simulink model "Monza_simulacion"  (R2023b)
settings: Solver=VariableStepAuto  StartTime=0.0  StopTime=20  RelTol=1e-3
values from neighbouring files (symbols this model uses):
  Ts = 0.005    [simulacion_monza_tfm.m]
libraries: slpidlib x2
settings Model: PauseTimes=20  Creator=christian  LastModifiedBy=Usuario
settings SolverCC: ZeroCrossAlgorithm=Adaptive  AlgebraicLoopSolver=TrustRegion
settings DataIOCC: ReturnWorkspaceOutputs=off
settings DebuggingCC: UnconnectedInputMsg=warning  UnconnectedOutputMsg=warning  UnconnectedLineMsg=warning  ArithmeticOperatorsInVariantConditions=warning
settings ModelReferenceCC: EnableRefExpFcnMdlSchedulingChecks=on
settings SFSimCC: SimUseLocalCustomCode=off  CustomCodeUndefinedFunction=UseInterfaceOnly
settings RTWCC: RTWUseLocalCustomCode=off

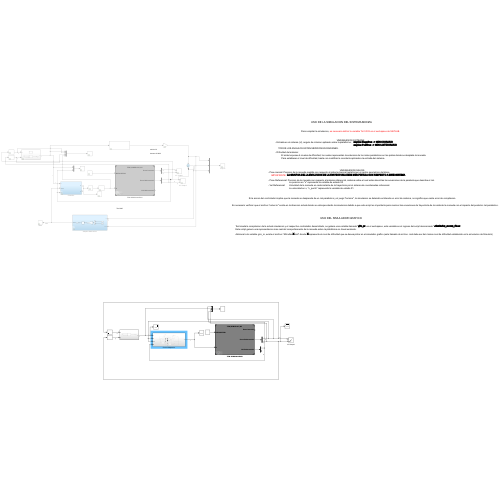
[thumbnail: Simulink's stored preview of the top-level diagram]
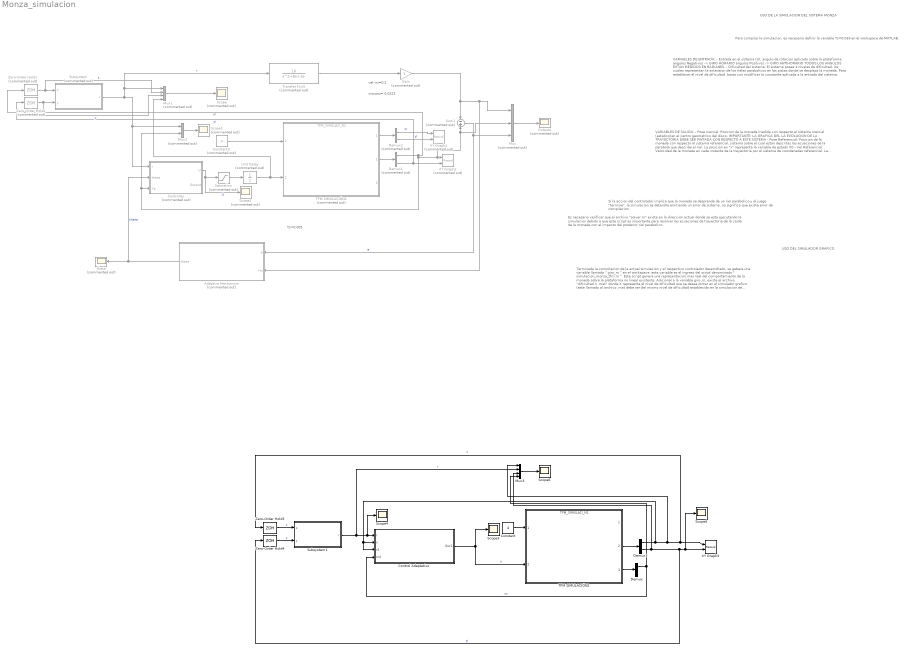
== system Monza_simulacion ==
  note: viscoso= 0.0223
  note: vel-ini=0.2
  note: Ts=0.005
  note: Es necesario verificar que el archivo "solver.m" exista en la direccion actual donde se esta ejecutando la simulacion debido a que este script es importante para resolver las ecuaciones de trayectoria de la caida de la moneda con el impacto del posterior riel parabolico.
  note: Si la accion del controlador implica que la moneda se desprenda de un riel parabolico y el juego "termine", la simulacion se detendra emitiendo un error de sistema, no significa que existe error de compilacion.
  note: Para compilar la simulacion, es necesario definir la variable Ts=0.033 en el workspace de MATLAB.
  note: VARIABLES DE ENTRADA:
      | - Entrada en el sistema (U), angulo de rotacion aplicado sobre la plataforma; angulos Negativos -> GIRO HORARIO
      | angulos Positivos -> GIRO ANTIHORARIO
      | TODOS LOS ANGULOS ESTAN MEDIDOS EN RADIANES.
      |
      | - Dificultad del sistema:
      | El sistema posee 4 niveles de dificultad, los cuales representan la extension de los rieles parabolicos en las pistas donde se desplaza la moneda.
      | Para establecer el nivel de dificultad, basta con modificar la constante aplicada a la entrada del sistema.
  note: USO DE LA SIMULACION DEL SISTEMA MONZA
  note: VARIABLES DE SALIDA:
      | - Pose inercial: Posicion de la moneda medida con respecto al sistema Inercial (estatico)en el centro geometrico del disco.
      | IMPORTANTE: LA GRAFICA DEL LA EVOLUCION DE LA TRAYECTORIA DEBE SER PINTADA CON RESPECTO A ESTE SISTEMA
      |
      | - Pose Referencial: Posicion de la moneda con respecto al sistema referencial, sistema sobre el cual estan descritas las ecuaciones de la parabola que describe el riel.
      | La posicion en "x" representa la variable de estado X0
      | - Vel Referencial: Velocidad de la moneda en cada instante de la trayectoria por el sistema de coordenadas referencial.
      | La velocidad en x, "x_punto" representa la variable de estado X1.
  note: USO DEL SIMULADOR GRAFICO
  note: Terminada la compilacion de la actual simulacion y el respectivo controlador desarrollado, se gebera una variable llamada " giro_m " en el workspace, esta variable es el ingreso del script denominado " simulacion_monza_tfm.m ".
      | Este script genera una representacion mas real del comportamiento de la moneda sobre la plataforma no lineal existente.
      |
      | Adicional a la variable giro_m, existe el archivo "dificultad X .mat" donde X representa el nivel de dificultad que se desea pintar en el simulador grafico (este llamado al archivo .mat debe ser del mismo nivel de dificultad establecido en la simulacion de Simulink)
  Adaptive Mechanism : Subsystem  Commented=on
  Constant : Constant  Value=4
  Constant3 : Constant  Commented=on  Value=4
  Control Adaptativo : Subsystem
  Controller : Subsystem  Commented=on
  Demux : Demux  Outputs=2
  Demux1 : Demux  Commented=on  Outputs=2
  Demux2 : Demux  Commented=on  Outputs=2
  Demux3 : Demux  Outputs=2
  Gain : Gain  Commented=on
  Mux : Mux  Commented=on  Inputs=3
  Mux1 : Mux  Commented=on
  Mux2 : Mux  Commented=on  Inputs=2
  Mux3 : Mux
  Outputs : Scope  Commented=on
  Saturation : Saturate  Commented=on  UpperLimit=0.3  LowerLimit=-0.3
  Scope : Scope  Commented=on
  Scope1 : Scope  Commented=on
  Scope2 : Scope  Commented=on
  Scope{3..6} (4 alike) : Scope
  Subsystem : Subsystem  Commented=on
  Subsystem1 : Subsystem
  Sum1 : Sum  Commented=on  Inputs=-|+
  TFM SIMULACIÓN1 : ModelReference  Commented=on  ModelNameDialog=TFM_SIMULACI_N1.slx  UsingDefaultArgumentValue=0,0  SimulationMode=Normal  ModelReferenceVersion=13.5  Gain=0.2  Gain2=0.0223
  TFM SIMULACIÓN2 : ModelReference  ModelNameDialog=TFM_SIMULACI_N1.slx  UsingDefaultArgumentValue=0,0  SimulationMode=Normal  ModelReferenceVersion=13.5  Gain=0.2  Gain2=0.0223
  Transfer Fcn5 : TransferFcn  Commented=on  Numerator=[16]  Denominator=[1 8 16]
  Unit Delay : UnitDelay  Commented=on  SampleTime=Ts  HasFrameUpgradeWarning=on
  XY Graph1 : Record  Commented=on  FileSettingsInternal="{\"entries\":[{\"content\":{\"excelSettings\":{\"content\":{},\"type\":\"Streamout.ExcelSettings\"}},\"type\":\"Streamout.FileSettingStorage\",\"uuid\":\"\"}],\"packageUris\":[\"http:\\/\\/schema.mathworks.com\\/mf0\\/streamout_blocks\\/R2020a\"],\"version\":\"1.0\"}"  Layout=[1 1]  SignalsInternal="{\"entries\":[{\"content\":{},\"type\":\"RecordBlkView.InputSignals\",\"uuid\":\"\"}],\"packageUris\":[\"http:\\/\\/schema.mathworks.com\\/mf0\\/streamout_blocks\\/R2020a\"],\"version\":\"1.0\"}"  VisualizationBindings="{\"xyplotplugin\":{\"info\":[{\"series\":[],\"subplotID\":1}]}}"  CompatibilityTag=XY  st=-1
  XY Graph2 : Record  Commented=on  FileSettingsInternal="{\"entries\":[{\"content\":{\"excelSettings\":{\"content\":{},\"type\":\"Streamout.ExcelSettings\"}},\"type\":\"Streamout.FileSettingStorage\",\"uuid\":\"\"}],\"packageUris\":[\"http:\\/\\/schema.mathworks.com\\/mf0\\/streamout_blocks\\/R2020a\"],\"version\":\"1.0\"}"  Layout=[1 1]  SignalsInternal="{\"entries\":[{\"content\":{},\"type\":\"RecordBlkView.InputSignals\",\"uuid\":\"\"}],\"packageUris\":[\"http:\\/\\/schema.mathworks.com\\/mf0\\/streamout_blocks\\/R2020a\"],\"version\":\"1.0\"}"  VisualizationBindings="{\"xyplotplugin\":{\"info\":[{\"series\":[],\"subplotID\":1}]}}"  CompatibilityTag=XY  st=-1
  XY Graph3 : Record  FileSettingsInternal="{\"entries\":[{\"content\":{\"excelSettings\":{\"content\":{},\"type\":\"Streamout.ExcelSettings\"}},\"type\":\"Streamout.FileSettingStorage\",\"uuid\":\"\"}],\"packageUris\":[\"http:\\/\\/schema.mathworks.com\\/mf0\\/streamout_blocks\\/R2020a\"],\"version\":\"1.0\"}"  Layout=[1 1]  SignalsInternal="{\"entries\":[{\"content\":{\"signals\":[{\"content\":{\"blockPath\":[],\"dimensions\":[1],\"domain\":\"\",\"lineColor\":\"#64d413\",\"port\":1,\"sid\":[\"\"],\"signalID\":6856,\"signalName\":\"x\"},\"type\":\"RecordBlkView.Signal\",\"uuid\":\"\"},{\"content\":{\"blockPath\":[],\"dimensions\":[1],\"domain\":\"\",\"lineColor\":\"#ff13a6\",\"port\":2,\"sid\":[\"\"],\"signalID\":6860,\"signalName\":\"yi\"},\"type\":\"RecordBlkView.Signal\",\"uuid\":\"\"}]},\"type\":\"RecordBlkView.InputSignals\",\"uuid\":\"\"}],\"packageUris\":[\"http:\\/\\/schema.mathworks.com\\/mf0\\/streamout_blocks\\/R2020a\"],\"version\":\"1.0\"}"  VisualizationBindings="{\"xyplotplugin\":{\"info\":[{\"series\":[],\"subplotID\":1}]}}"  CompatibilityTag=XY  st=-1
  Zero-Order Hold1 : ZeroOrderHold  Commented=on  SampleTime=Ts
  Zero-Order Hold2 : ZeroOrderHold  Commented=on  SampleTime=Ts
  Zero-Order Hold3 : ZeroOrderHold  SampleTime=Ts
  Zero-Order Hold4 : ZeroOrderHold  SampleTime=Ts
  theta : Scope  Commented=on
  wires:
  Constant3/1 -> TFM SIMULACIÓN1/1
  Adaptive Mechanism/1(theta) -> Controller/2(theta), theta/1  "theta"
  Mux/1 -> Outputs/1
  Controller/1(U) -> Scope2/1, Saturation/1  "U"
  Sum1/1 -> Adaptive Mechanism/1(e), Mux/3  "e"
  Subsystem/1(r) -> Transfer Fcn5/1, Mux1/1, Controller/1(r), Mux2/1  "r"
  TFM SIMULACIÓN1/2 -> Demux1/1
  Demux1/1 -> Zero-Order Hold1/1, Mux2/2, Controller/3(Yp), Mux/2, Sum1/2, XY Graph2/1  "xr"
  Demux1/2 -> Zero-Order Hold2/1, XY Graph2/2  "yi"
  Mux1/1 -> Scope/1
  Zero-Order Hold1/1 -> Mux1/2, Subsystem/1(x)  "x"
  Zero-Order Hold2/1 -> Mux1/3, Subsystem/2(y)  "y"
  Mux2/1 -> Scope1/1
  Unit Delay/1 -> Mux1/4, TFM SIMULACIÓN1/2
  Saturation/1 -> Unit Delay/1
  TFM SIMULACIÓN1/1 -> Demux2/1
  Demux2/2 -> XY Graph1/2  "yi"
  Demux2/1 -> XY Graph1/1  "xr"
  Gain/1 -> Adaptive Mechanism/2(Ym), Mux/1, Sum1/1
  Demux3/1 -> Mux3/1, Zero-Order Hold3/1, XY Graph3/1, Control Adaptativo/3(x1), Control Adaptativo/2(x)  "x"
  Zero-Order Hold3/1 -> Subsystem1/1(x)  "x"
  Zero-Order Hold4/1 -> Subsystem1/2(y)  "y"
  TFM SIMULACIÓN2/2 -> Demux3/1
  Demux3/2 -> Mux3/3, Zero-Order Hold4/1, Scope5/1, XY Graph3/2  "yi"
  Constant/1 -> TFM SIMULACIÓN2/1
  Transfer Fcn5/1 -> Gain/1
  TFM SIMULACIÓN2/3 -> Demux/1
  Subsystem1/1(r) -> Mux3/2, Scope4/1, Control Adaptativo/1(r)  "r"
  Demux/1 -> Mux3/4, Control Adaptativo/4(In4)  "vx"
  Control Adaptativo/1(Out1) -> TFM SIMULACIÓN2/2, Scope3/1  "u"
  Mux3/1 -> Scope6/1

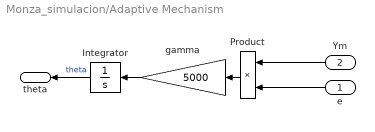
== system Monza_simulacion/Adaptive Mechanism ==
  e : Inport
  Ym : Inport  Port=2
  Integrator : Integrator  InitialCondition=1
  Product : Product
  gamma : Gain  Gain=5000
  theta : Outport  VectorParamsAs1DForOutWhenUnconnected=off
  wires:
  Integrator/1 -> theta/1  "theta"
  gamma/1 -> Integrator/1
  Product/1 -> gamma/1
  Ym/1 -> Product/1
  e/1 -> Product/2

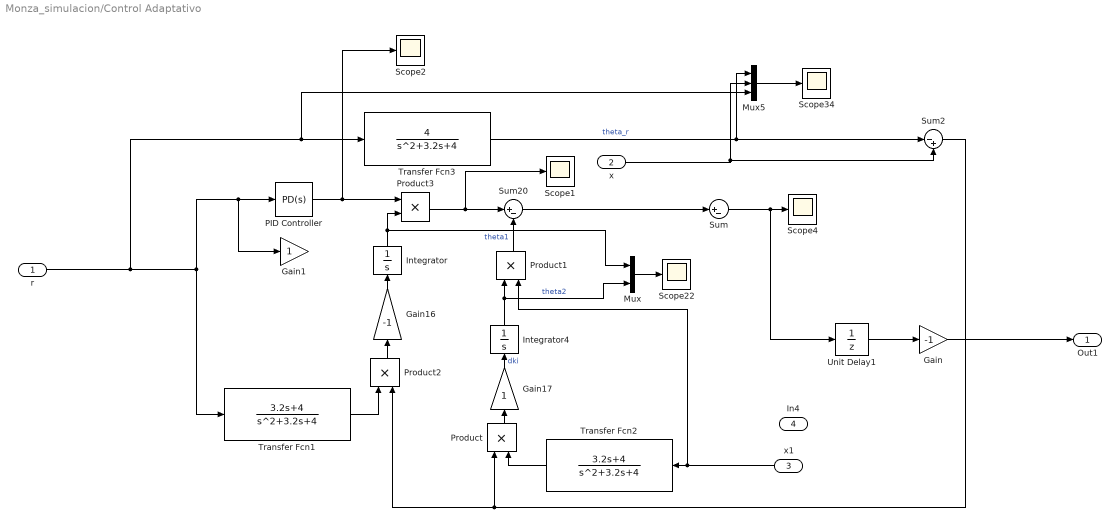
== system Monza_simulacion/Control Adaptativo ==
  r : Inport
  x : Inport  Port=2
  x1 : Inport  Port=3
  In4 : Inport  Port=4
  Gain : Gain  Gain=-1
  Gain1 : Gain
  Gain16 : Gain  Gain=-1
  Gain17 : Gain
  Integrator : Integrator  InitialCondition=1
  Integrator4 : Integrator  InitialCondition=1
  Mux : Mux  Inputs=2
  Mux5 : Mux  Inputs=3
  PID Controller : slpidlib/PID Controller  Controller=PD  Form=Parallel  TimeDomain=Continuous-time  UseExternalTs=off  SampleTime=-1  IntegratorMethod=Forward Euler  FilterMethod=Forward Euler  ControllerParametersSource=internal  P=0.2  I=1  UseKiTs=off  D=0.05  N=10  UseFilter=on  TunerSelectOption=Transfer Function Based (PID Tuner App)  InitialConditionSource=internal  InitialConditionForIntegrator=0  InitialConditionForFilter=0  DifferentiatorICPrevScaledInput=0  ExternalReset=none  TrackingMode=off  Kt=1  LimitOutput=off  SatLimitsSource=internal  UpperSaturationLimit=inf  LowerSaturationLimit=-inf  LinearizeAsGain=on  AntiWindupMode=none  Kb=1  LimitIntegrator=off  UpperIntegratorSaturationLimit=inf  LowerIntegratorSaturationLimit=-inf  POutMin=[]  POutMax=[]  IOutMin=[]  IOutMax=[]  DOutMin=[]  DOutMax=[]  NOutMin=[]  NOutMax=[]  SumOutMin=[]  SumOutMax=[]  SaturationOutMin=[]  SaturationOutMax=[]  PParamMin=[]  PParamMax=[]  IParamMin=[]  IParamMax=[]  DParamMin=[]  DParamMax=[]  NParamMin=[]  NParamMax=[]  KbParamMin=[]  KbParamMax=[]  KtParamMin=[]  KtParamMax=[]  KbOutMin=[]  KbOutMax=[]  KtOutMin=[]  KtOutMax=[]  IntegratorOutMin=[]  IntegratorOutMax=[]  FilterOutMin=[]  FilterOutMax=[]  SumI1OutMin=[]  SumI1OutMax=[]  SumI2OutMin=[]  SumI2OutMax=[]  SumI3OutMin=[]  SumI3OutMax=[]  SumI4OutMin=[]  SumI4OutMax=[]  SumDOutMin=[]  SumDOutMax=[]  DifferentiatorOutMin=[]  DifferentiatorOutMax=[]  FilterDiffOutCoefMin=[]  FilterDiffOutCoefMax=[]  ReciprocalOutMin=[]  ReciprocalOutMax=[]  SumDenOutMin=[]  SumDenOutMax=[]  SumNumOutMin=[]  SumNumOutMax=[]  DivideOutMin=[]  DivideOutMax=[]  UdiffTsProdOutMin=[]  UdiffTsProdOutMax=[]  NTsProdOutMin=[]  NTsProdOutMax=[]  UintegralTsProdOutMin=[]  UintegralTsProdOutMax=[]  UngainTsProdOutMin=[]  UngainTsProdOutMax=[]  ClampingZeroOutDataTypeStr=Inherit: Inherit via back propagation  ClampingZeroOutMin=[]  ClampingZeroOutMax=[]  FilterDenConstantOutDataTypeStr=Inherit: Inherit via back propagation  FilterDenConstantOutMin=[]  FilterDenConstantOutMax=[]  PCopyOutDataTypeStr=Inherit: Inherit via back propagation  PCopyOutMin=[]  PCopyOutMax=[]  NCopyOutDataTypeStr=Inherit: Inherit via back propagation  NCopyOutMin=[]  NCopyOutMax=[]  IntegratorContinuousStateAttributes=''  IntegratorStateMustResolveToSignalObject=off  IntegratorRTWStateStorageClass=Auto  FilterContinuousStateAttributes=''  FilterStateMustResolveToSignalObject=off  FilterRTWStateStorageClass=Auto  ParallelPVariant=InternalParameters  IdealPVariant=Disabled  IVariant=Disabled  DVariant=InternalParameters  IntegratorVariant=Disabled  SatVariant=Disabled  AWVariant=Disabled  PCopyVariant=Disabled  TRVariant=Disabled  FdbkBlocksVariant=Forward  IdealPFdbkVariant=Disabled  SatFdbkVariant=Disabled  DerivativeFilterVariant=ContFilter  NVariant=InternalParameters  NCopyVariant=Disabled  FilterICVariant=InternalICsFilter  IntegratorICVariant=Disabled  ExternalResetVariant=Disabled  TRSumVariant=Passthrough  SumFdbkVariant=Disabled  SumVariant=Sum_PD  TsampFilterVariant=InternalTs  TsampNgainVariant=Passthrough  TsampIntegralVariant=Disabled_SignalSpec  ExternalSaturationOutDataTypeStr=Inherit: Same as second input
  Product{,1..3} (4 alike) : Product
  Scope{1..2,4,22,34} (5 alike) : Scope
  Sum : Sum  Inputs=|+-
  Sum2 : Sum  Inputs=|-+
  Sum20 : Sum  Inputs=|+-
  Transfer Fcn1 : TransferFcn  Numerator=[3.2 4]  Denominator=[1 3.2 4]
  Transfer Fcn2 : TransferFcn  Numerator=[3.2 4]  Denominator=[1 3.2 4]
  Transfer Fcn3 : TransferFcn  Numerator=[4]  Denominator=[1 3.2 4]
  Unit Delay1 : UnitDelay  SampleTime=Ts  HasFrameUpgradeWarning=on
  Out1 : Outport
  wires:
  r/1 -> Transfer Fcn3/1, Mux5/3, Transfer Fcn1/1, Gain1/1, PID Controller/1
  x1/1 -> Transfer Fcn2/1, Product1/2
  x/1 -> Mux5/2, Sum2/2
  Product1/1 -> Sum20/2
  Gain16/1 -> Integrator/1
  Mux5/1 -> Scope34/1
  Product3/1 -> Scope1/1, Sum20/1
  Transfer Fcn3/1 -> Mux5/1, Sum2/1  "theta_r"
  Product2/1 -> Gain16/1
  Integrator/1 -> Product3/2, Mux/1  "theta1"
  Integrator4/1 -> Product1/1, Mux/2  "theta2"
  Transfer Fcn1/1 -> Product2/1
  Product/1 -> Gain17/1
  Gain17/1 -> Integrator4/1  "dki"
  Sum/1 -> Scope4/1, Unit Delay1/1
  Transfer Fcn2/1 -> Product/2
  Sum2/1 -> Product/1, Product2/2
  Unit Delay1/1 -> Gain/1
  Gain/1 -> Out1/1
  Mux/1 -> Scope22/1
  PID Controller/1 -> Product3/1, Scope2/1
  Sum20/1 -> Sum/1

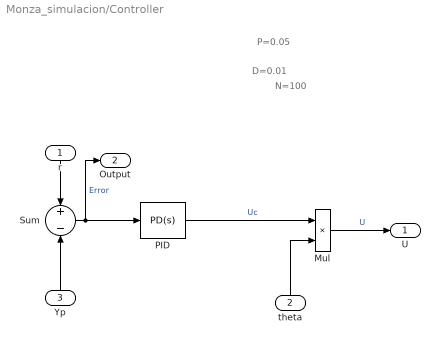
== system Monza_simulacion/Controller ==
  note: N=100
  note: D=0.01
  note: P=0.05
  r : Inport
  theta : Inport  Port=2
  Yp : Inport  Port=3
  Mul : Product
  PID : slpidlib/PID Controller  Controller=PD  Form=Parallel  TimeDomain=Continuous-time  UseExternalTs=off  SampleTime=1  IntegratorMethod=Forward Euler  FilterMethod=Forward Euler  ControllerParametersSource=internal  P=0.05  I=1  UseKiTs=off  D=0.01  N=100  UseFilter=on  TunerSelectOption=Transfer Function Based (PID Tuner App)  InitialConditionSource=internal  InitialConditionForIntegrator=0  InitialConditionForFilter=0  DifferentiatorICPrevScaledInput=0  ExternalReset=none  TrackingMode=off  Kt=1  LimitOutput=off  SatLimitsSource=internal  UpperSaturationLimit=inf  LowerSaturationLimit=-inf  LinearizeAsGain=on  AntiWindupMode=none  Kb=1  LimitIntegrator=off  UpperIntegratorSaturationLimit=inf  LowerIntegratorSaturationLimit=-inf  POutMin=[]  POutMax=[]  IOutMin=[]  IOutMax=[]  DOutMin=[]  DOutMax=[]  NOutMin=[]  NOutMax=[]  SumOutMin=[]  SumOutMax=[]  SaturationOutMin=[]  SaturationOutMax=[]  PParamMin=[]  PParamMax=[]  IParamMin=[]  IParamMax=[]  DParamMin=[]  DParamMax=[]  NParamMin=[]  NParamMax=[]  KbParamMin=[]  KbParamMax=[]  KtParamMin=[]  KtParamMax=[]  KbOutMin=[]  KbOutMax=[]  KtOutMin=[]  KtOutMax=[]  IntegratorOutMin=[]  IntegratorOutMax=[]  FilterOutMin=[]  FilterOutMax=[]  SumI1OutMin=[]  SumI1OutMax=[]  SumI2OutMin=[]  SumI2OutMax=[]  SumI3OutMin=[]  SumI3OutMax=[]  SumI4OutMin=[]  SumI4OutMax=[]  SumDOutMin=[]  SumDOutMax=[]  DifferentiatorOutMin=[]  DifferentiatorOutMax=[]  FilterDiffOutCoefMin=[]  FilterDiffOutCoefMax=[]  ReciprocalOutMin=[]  ReciprocalOutMax=[]  SumDenOutMin=[]  SumDenOutMax=[]  SumNumOutMin=[]  SumNumOutMax=[]  DivideOutMin=[]  DivideOutMax=[]  UdiffTsProdOutMin=[]  UdiffTsProdOutMax=[]  NTsProdOutMin=[]  NTsProdOutMax=[]  UintegralTsProdOutMin=[]  UintegralTsProdOutMax=[]  UngainTsProdOutMin=[]  UngainTsProdOutMax=[]  ClampingZeroOutDataTypeStr=Inherit: Inherit via back propagation  ClampingZeroOutMin=[]  ClampingZeroOutMax=[]  FilterDenConstantOutDataTypeStr=Inherit: Inherit via back propagation  FilterDenConstantOutMin=[]  FilterDenConstantOutMax=[]  PCopyOutDataTypeStr=Inherit: Inherit via back propagation  PCopyOutMin=[]  PCopyOutMax=[]  NCopyOutDataTypeStr=Inherit: Inherit via back propagation  NCopyOutMin=[]  NCopyOutMax=[]  IntegratorContinuousStateAttributes=''  IntegratorStateMustResolveToSignalObject=off  IntegratorRTWStateStorageClass=Auto  FilterContinuousStateAttributes=''  FilterStateMustResolveToSignalObject=off  FilterRTWStateStorageClass=Auto  ParallelPVariant=InternalParameters  IdealPVariant=Disabled  IVariant=Disabled  DVariant=InternalParameters  IntegratorVariant=Disabled  SatVariant=Disabled  AWVariant=Disabled  PCopyVariant=Disabled  TRVariant=Disabled  FdbkBlocksVariant=Forward  IdealPFdbkVariant=Disabled  SatFdbkVariant=Disabled  DerivativeFilterVariant=ContFilter  NVariant=InternalParameters  NCopyVariant=Disabled  FilterICVariant=InternalICsFilter  IntegratorICVariant=Disabled  ExternalResetVariant=Disabled  TRSumVariant=Passthrough  SumFdbkVariant=Disabled  SumVariant=Sum_PD  TsampFilterVariant=InternalTs  TsampNgainVariant=Passthrough  TsampIntegralVariant=Disabled_SignalSpec  ExternalSaturationOutDataTypeStr=Inherit: Same as second input
  Sum : Sum  Inputs=+|-
  U : Outport  VectorParamsAs1DForOutWhenUnconnected=off
  Output : Outport  Port=2
  wires:
  theta/1 -> Mul/2
  r/1 -> Sum/1
  Yp/1 -> Sum/2
  PID/1 -> Mul/1  "Uc"
  Sum/1 -> PID/1, Output/1  "Error"
  Mul/1 -> U/1  "U"

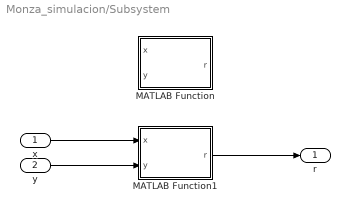
== system Monza_simulacion/Subsystem ==
  x : Inport
  y : Inport  Port=2
  MATLAB Function : MATLAB Function  TreatAsAtomicUnit=on
  MATLAB Function1 : MATLAB Function  TreatAsAtomicUnit=on
  r : Outport
  wires:
  y/1 -> MATLAB Function1/2(y)
  x/1 -> MATLAB Function1/1(x)
  MATLAB Function1/1(r) -> r/1

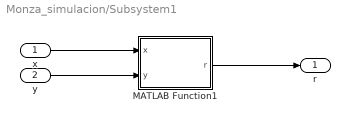
== system Monza_simulacion/Subsystem1 ==
  x : Inport
  y : Inport  Port=2
  MATLAB Function1 : MATLAB Function  TreatAsAtomicUnit=on
  r : Outport
  wires:
  y/1 -> MATLAB Function1/2(y)
  x/1 -> MATLAB Function1/1(x)
  MATLAB Function1/1(r) -> r/1

== matlab function Monza_simulacion/Subsystem/MATLAB Function ==
  data: x input; r output; y input
function r = fcn(x,y)
%#codegen
r=0;
if(x>-0.02554 && y>-0.16035 )

    r=-0.0256;
end
if(x>-0.05409 && y>-0.11585)

    r=-0.055;
end
if(x<0.04406 && y>-0.06961)

    r=0.045;
end
if(x>-0.04847 && y >-0.02411)

    r=-0.05;
end
if(x<0.04969 && y>0.02154)

    r=0.05;
end
if(x>-0.04758 && y>0.06799)

    r=-0.063;
end
if(x<0.06211 && y>0.112)

    r=0.063;
end

== matlab function Monza_simulacion/Subsystem1/MATLAB Function1 ==
  data: x input; r output; y input
function r = fcn(x,y)
%#codegen
r=0;
if(x>-0.0256 && y>=-0.161 )

    r=-0.0256;
end
if(x>-0.11 && y>=-0.13 )

    r=-0.108;
end
if(x<0.132 && y>=-0.09  )

    r=0.1318;
end
if(x>-0.149 && y>=-0.045 )

    r=-0.14851;
end
if(x<0.1425 && y>=0.005 )

    r=0.14224;
end
if(x>-0.1425 && y>=0.05 )

    r=-0.14224;
end
if(x<0.12394 && y>=0.10)

   r=0.124;
end

== matlab function Monza_simulacion/Subsystem/MATLAB Function1 ==
  data: x input; r output; y input
function r = fcn(x,y)
%#codegen
r=0;
if(x>-0.0256 && y>-0.161 )

    r=-0.0256;
end
if(x>-0.11 && y>-0.13)

    r=-0.108;
end
if(x<0.132 && y>-0.082)

    r=0.1318;
end
if(x>-0.149 && y>-0.035)

    r=-0.14851;
end
if(x<0.1425 && y>0.010)

    r=0.14224;
end
if(x>-0.1425 && y>0.05)

    r=-0.14224;
end
if(x<0.12394 && y>0.10)

    r=0.124;
end
